simulink library "sm_car_lib"  (R2024a)
settings: Solver=VariableStepAuto  StartTime=0.0  StopTime=10.0  RelTol=1e-3
undefined symbols (not defined in the file or in its folder): acc_theta, accel_ramp_rate, circ_out, clr_upr, Control, hp1, hp2, hp3, hp_in_f_ua, hp_in_r_ua, hp_la_out, hp_ua_out, Init, Newton, opc_upr, radius_upr, Raphson, RDF_Rough_Road, rhs_hp, Scene, ShaftF, ShaftR, Vehicle, Visual, X, Y, Z
libraries: sm_lib x117, $bdroot x97, nesl_utility x36, simulink x17, fl_lib x6, sharedtransformsys x3, Brakes_Elements x2, Driver_Gamepad_Xbox x2, Multibody_Parts_Lib x2, sm_car_scene_track_mallory_park_obstacle x2, Testrig_4Post_Inputs x2, Aero_Coefficients x1
(part 4 of 7)

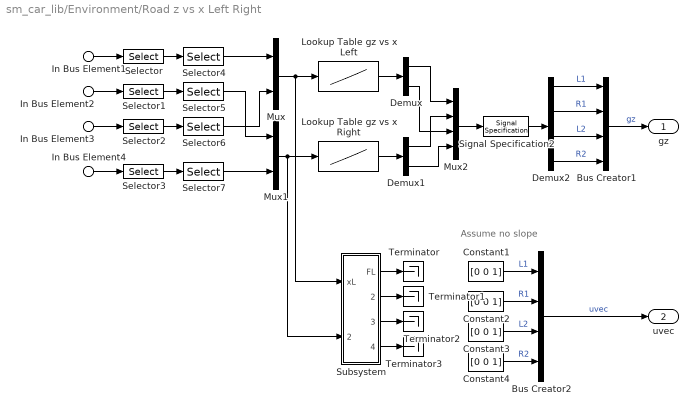
== system sm_car_lib/Environment/Road z vs x Left Right ==
  note: Assume no slope
  In Bus Element1 : Inport  PortName=Chassis  Element=WhlL1.xyz
  In Bus Element2 : Inport  PortName=Chassis  Element=WhlR1.xyz
  In Bus Element3 : Inport  PortName=Chassis  Element=WhlL2.xyz
  In Bus Element4 : Inport  PortName=Chassis  Element=WhlR2.xyz
  Bus Creator1 : BusCreator  Inputs=4
  Bus Creator2 : BusCreator  Inputs=4
  Constant{1..4} (4 alike) : Constant  Value=[0 0 1]
  Demux : Demux  Outputs=2
  Demux1 : Demux  Outputs=2
  Demux2 : Demux
  Lookup Table gz vs x Left : Lookup_n-D  NumberOfTableDimensions=1  BreakpointsForDimension1=dist_x_l  Table=height_z_l  InternalRulePriority=Speed  RndMeth=Simplest
  Lookup Table gz vs x Right : Lookup_n-D  NumberOfTableDimensions=1  BreakpointsForDimension1=dist_x_r  Table=height_z_r  InternalRulePriority=Speed  RndMeth=Simplest
  Mux : Mux  Inputs=2
  Mux1 : Mux  Inputs=2
  Mux2 : Mux
  Selector{,1..3} (4 alike) : Selector  InputPortWidth=3  IndexOptions=Index vector (dialog)  Indices=[1 2]  OutputSizes=1
  Selector{4..7} (4 alike) : Selector  InputPortWidth=2  IndexOptions=Index vector (dialog)  Indices=1  OutputSizes=1
  Signal Specification2 : SignalSpecification  Unit=m
  Subsystem : Subsystem
  Terminator{,1..3} (4 alike) : Terminator
  gz : Outport  VectorParamsAs1DForOutWhenUnconnected=off
  uvec : Outport  Port=2  VectorParamsAs1DForOutWhenUnconnected=off
  wires:
  Signal Specification2/1 -> Demux2/1
  In Bus Element3/1 -> Selector2/1
  In Bus Element1/1 -> Selector/1
  In Bus Element2/1 -> Selector1/1
  In Bus Element4/1 -> Selector3/1
  Selector/1 -> Selector4/1
  Selector1/1 -> Selector5/1
  Selector2/1 -> Selector6/1
  Selector3/1 -> Selector7/1
  Selector7/1 -> Mux1/2
  Selector6/1 -> Mux/2
  Selector5/1 -> Mux1/1
  Selector4/1 -> Mux/1
  Lookup Table gz vs x Right/1 -> Demux1/1
  Lookup Table gz vs x Left/1 -> Demux/1
  Demux/1 -> Mux2/1
  Demux1/1 -> Mux2/2
  Demux/2 -> Mux2/3
  Demux1/2 -> Mux2/4
  Mux2/1 -> Signal Specification2/1
  Mux1/1 -> Subsystem/2(xR), Lookup Table gz vs x Right/1
  Mux/1 -> Subsystem/1(xL), Lookup Table gz vs x Left/1
  Demux2/1 -> Bus Creator1/1  "L1"
  Demux2/2 -> Bus Creator1/2  "R1"
  Demux2/3 -> Bus Creator1/3  "L2"
  Demux2/4 -> Bus Creator1/4  "R2"
  Bus Creator1/1 -> gz/1  "gz"
  Constant1/1 -> Bus Creator2/1  "L1"
  Constant3/1 -> Bus Creator2/3  "L2"
  Constant2/1 -> Bus Creator2/2  "R1"
  Bus Creator2/1 -> uvec/1  "uvec"
  Constant4/1 -> Bus Creator2/4  "R2"
  Subsystem/1(FL) -> Terminator/1
  Subsystem/4(RR) -> Terminator3/1
  Subsystem/2(FR) -> Terminator1/1
  Subsystem/3(RL) -> Terminator2/1

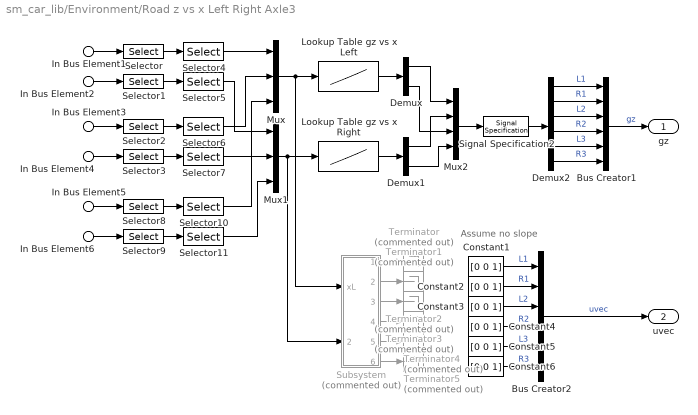
== system sm_car_lib/Environment/Road z vs x Left Right Axle3 ==
  note: Assume no slope
  In Bus Element1 : Inport  PortName=Chassis  Element=WhlL1.xyz
  In Bus Element2 : Inport  PortName=Chassis  Element=WhlR1.xyz
  In Bus Element3 : Inport  PortName=Chassis  Element=WhlL2.xyz
  In Bus Element4 : Inport  PortName=Chassis  Element=WhlR2.xyz
  In Bus Element5 : Inport  PortName=Chassis  Element=WhlL3.xyz
  In Bus Element6 : Inport  PortName=Chassis  Element=WhlR3.xyz
  Bus Creator1 : BusCreator  Inputs=6
  Bus Creator2 : BusCreator  Inputs=6
  Constant{1..6} (6 alike) : Constant  Value=[0 0 1]
  Demux : Demux  Outputs=2
  Demux1 : Demux  Outputs=2
  Demux2 : Demux  Outputs=6
  Lookup Table gz vs x Left : Lookup_n-D  NumberOfTableDimensions=1  BreakpointsForDimension1=dist_x_l  Table=height_z_l  InternalRulePriority=Speed  RndMeth=Simplest
  Lookup Table gz vs x Right : Lookup_n-D  NumberOfTableDimensions=1  BreakpointsForDimension1=dist_x_r  Table=height_z_r  InternalRulePriority=Speed  RndMeth=Simplest
  Mux : Mux  Inputs=3
  Mux1 : Mux  Inputs=3
  Mux2 : Mux
  Selector{,1..3,8..9} (6 alike) : Selector  InputPortWidth=3  IndexOptions=Index vector (dialog)  Indices=[1 2]  OutputSizes=1
  Selector{4..7,10..11} (6 alike) : Selector  InputPortWidth=2  IndexOptions=Index vector (dialog)  Indices=1  OutputSizes=1
  Signal Specification2 : SignalSpecification  Unit=m
  Subsystem : Subsystem  Commented=on
  Terminator{,1..5} (6 alike) : Terminator  Commented=on
  gz : Outport  VectorParamsAs1DForOutWhenUnconnected=off
  uvec : Outport  Port=2  VectorParamsAs1DForOutWhenUnconnected=off
  wires:
  Subsystem/3(L2) -> Terminator2/1
  Subsystem/2(R1) -> Terminator1/1
  Subsystem/4(R2) -> Terminator3/1
  Subsystem/1(L1) -> Terminator/1
  Constant4/1 -> Bus Creator2/4  "R2"
  Bus Creator2/1 -> uvec/1  "uvec"
  Constant2/1 -> Bus Creator2/2  "R1"
  Constant3/1 -> Bus Creator2/3  "L2"
  Constant1/1 -> Bus Creator2/1  "L1"
  Bus Creator1/1 -> gz/1  "gz"
  Demux2/4 -> Bus Creator1/4  "R2"
  Demux2/3 -> Bus Creator1/3  "L2"
  Demux2/2 -> Bus Creator1/2  "R1"
  Demux2/1 -> Bus Creator1/1  "L1"
  Mux/1 -> Lookup Table gz vs x Left/1, Subsystem/1(xL)
  Mux1/1 -> Lookup Table gz vs x Right/1, Subsystem/2(xR)
  Mux2/1 -> Signal Specification2/1
  Demux1/2 -> Mux2/4
  Demux/2 -> Mux2/3
  Demux1/1 -> Mux2/2
  Demux/1 -> Mux2/1
  Lookup Table gz vs x Left/1 -> Demux/1
  Lookup Table gz vs x Right/1 -> Demux1/1
  Selector4/1 -> Mux/1
  Selector5/1 -> Mux1/1
  Selector6/1 -> Mux/2
  Selector7/1 -> Mux1/2
  Selector3/1 -> Selector7/1
  Selector2/1 -> Selector6/1
  Selector1/1 -> Selector5/1
  Selector/1 -> Selector4/1
  In Bus Element4/1 -> Selector3/1
  In Bus Element2/1 -> Selector1/1
  In Bus Element1/1 -> Selector/1
  In Bus Element3/1 -> Selector2/1
  Signal Specification2/1 -> Demux2/1
  In Bus Element5/1 -> Selector8/1
  In Bus Element6/1 -> Selector9/1
  Selector8/1 -> Selector10/1
  Selector9/1 -> Selector11/1
  Selector10/1 -> Mux/3
  Selector11/1 -> Mux1/3
  Demux2/5 -> Bus Creator1/5  "L3"
  Demux2/6 -> Bus Creator1/6  "R3"
  Constant5/1 -> Bus Creator2/5  "L3"
  Constant6/1 -> Bus Creator2/6  "R3"
  Subsystem/5(L3) -> Terminator4/1
  Subsystem/6(R3) -> Terminator5/1

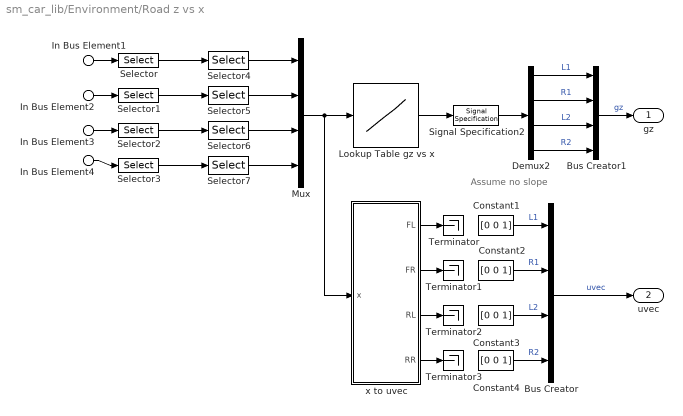
== system sm_car_lib/Environment/Road z vs x  ==
  note: Assume no slope
  In Bus Element1 : Inport  PortName=Chassis  Element=WhlL1.xyz
  In Bus Element2 : Inport  PortName=Chassis  Element=WhlR1.xyz
  In Bus Element3 : Inport  PortName=Chassis  Element=WhlL2.xyz
  In Bus Element4 : Inport  PortName=Chassis  Element=WhlR2.xyz
  Bus Creator : BusCreator  Inputs=4
  Bus Creator1 : BusCreator  Inputs=4
  Constant{1..4} (4 alike) : Constant  Value=[0 0 1]
  Demux2 : Demux
  Lookup Table gz vs x : Lookup_n-D  NumberOfTableDimensions=1  BreakpointsForDimension1=dist_x  Table=height_z  InternalRulePriority=Speed  RndMeth=Simplest
  Mux : Mux
  Selector{,1..3} (4 alike) : Selector  InputPortWidth=3  IndexOptions=Index vector (dialog)  Indices=[1 2]  OutputSizes=1
  Selector{4..7} (4 alike) : Selector  InputPortWidth=2  IndexOptions=Index vector (dialog)  Indices=1  OutputSizes=1
  Signal Specification2 : SignalSpecification  Unit=m
  Terminator{,1..3} (4 alike) : Terminator
  x to uvec : Subsystem
  gz : Outport  VectorParamsAs1DForOutWhenUnconnected=off
  uvec : Outport  Port=2  VectorParamsAs1DForOutWhenUnconnected=off
  wires:
  Lookup Table gz vs x/1 -> Signal Specification2/1
  Mux/1 -> x to uvec/1(x), Lookup Table gz vs x/1
  Selector4/1 -> Mux/1
  Selector5/1 -> Mux/2
  Selector6/1 -> Mux/3
  Selector7/1 -> Mux/4
  Selector3/1 -> Selector7/1
  Selector2/1 -> Selector6/1
  Selector1/1 -> Selector5/1
  Selector/1 -> Selector4/1
  In Bus Element4/1 -> Selector3/1
  In Bus Element2/1 -> Selector1/1
  In Bus Element1/1 -> Selector/1
  In Bus Element3/1 -> Selector2/1
  Demux2/3 -> Bus Creator1/3  "L2"
  Signal Specification2/1 -> Demux2/1
  Demux2/2 -> Bus Creator1/2  "R1"
  Demux2/1 -> Bus Creator1/1  "L1"
  Demux2/4 -> Bus Creator1/4  "R2"
  Bus Creator1/1 -> gz/1  "gz"
  Bus Creator/1 -> uvec/1  "uvec"
  Constant1/1 -> Bus Creator/1  "L1"
  x to uvec/1(FL) -> Terminator/1
  x to uvec/2(FR) -> Terminator1/1
  x to uvec/3(RL) -> Terminator2/1
  x to uvec/4(RR) -> Terminator3/1
  Constant2/1 -> Bus Creator/2  "R1"
  Constant3/1 -> Bus Creator/3  "L2"
  Constant4/1 -> Bus Creator/4  "R2"

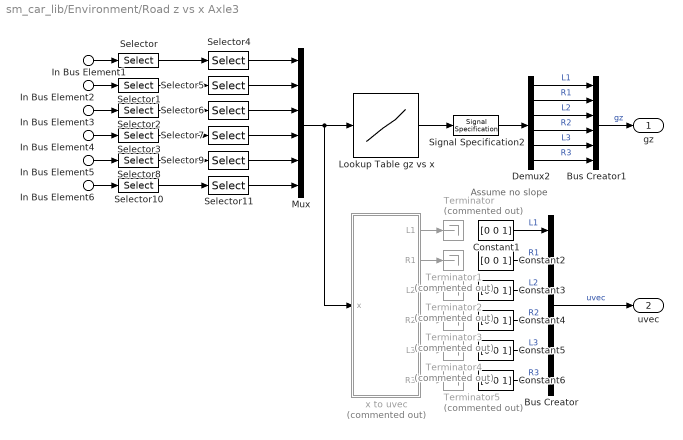
== system sm_car_lib/Environment/Road z vs x Axle3 ==
  note: Assume no slope
  In Bus Element1 : Inport  PortName=Chassis  Element=WhlL1.xyz
  In Bus Element2 : Inport  PortName=Chassis  Element=WhlR1.xyz
  In Bus Element3 : Inport  PortName=Chassis  Element=WhlL2.xyz
  In Bus Element4 : Inport  PortName=Chassis  Element=WhlR2.xyz
  In Bus Element5 : Inport  PortName=Chassis  Element=WhlL3.xyz
  In Bus Element6 : Inport  PortName=Chassis  Element=WhlR3.xyz
  Bus Creator : BusCreator  Inputs=6
  Bus Creator1 : BusCreator  Inputs=6
  Constant{1..6} (6 alike) : Constant  Value=[0 0 1]
  Demux2 : Demux  Outputs=6
  Lookup Table gz vs x : Lookup_n-D  NumberOfTableDimensions=1  BreakpointsForDimension1=dist_x  Table=height_z  InternalRulePriority=Speed  RndMeth=Simplest
  Mux : Mux  Inputs=6
  Selector{,1..3,8,10} (6 alike) : Selector  InputPortWidth=3  IndexOptions=Index vector (dialog)  Indices=[1 2]  OutputSizes=1
  Selector{4..7,9,11} (6 alike) : Selector  InputPortWidth=2  IndexOptions=Index vector (dialog)  Indices=1  OutputSizes=1
  Signal Specification2 : SignalSpecification  Unit=m
  Terminator{,1..5} (6 alike) : Terminator  Commented=on
  x to uvec : Subsystem  Commented=on
  gz : Outport  VectorParamsAs1DForOutWhenUnconnected=off
  uvec : Outport  Port=2  VectorParamsAs1DForOutWhenUnconnected=off
  wires:
  Constant4/1 -> Bus Creator/4  "R2"
  Constant3/1 -> Bus Creator/3  "L2"
  Constant2/1 -> Bus Creator/2  "R1"
  x to uvec/4(R2) -> Terminator3/1
  x to uvec/3(L2) -> Terminator2/1
  x to uvec/2(R1) -> Terminator1/1
  x to uvec/1(L1) -> Terminator/1
  Constant1/1 -> Bus Creator/1  "L1"
  Bus Creator/1 -> uvec/1  "uvec"
  Bus Creator1/1 -> gz/1  "gz"
  Demux2/4 -> Bus Creator1/4  "R2"
  Demux2/1 -> Bus Creator1/1  "L1"
  Demux2/2 -> Bus Creator1/2  "R1"
  Signal Specification2/1 -> Demux2/1
  Demux2/3 -> Bus Creator1/3  "L2"
  In Bus Element3/1 -> Selector2/1
  In Bus Element1/1 -> Selector/1
  In Bus Element2/1 -> Selector1/1
  In Bus Element4/1 -> Selector3/1
  Selector/1 -> Selector4/1
  Selector1/1 -> Selector5/1
  Selector2/1 -> Selector6/1
  Selector3/1 -> Selector7/1
  Selector7/1 -> Mux/4
  Selector6/1 -> Mux/3
  Selector5/1 -> Mux/2
  Selector4/1 -> Mux/1
  Mux/1 -> Lookup Table gz vs x/1, x to uvec/1(x)
  Lookup Table gz vs x/1 -> Signal Specification2/1
  Selector8/1 -> Selector9/1
  In Bus Element5/1 -> Selector8/1
  Selector9/1 -> Mux/5
  Selector11/1 -> Mux/6
  In Bus Element6/1 -> Selector10/1
  Selector10/1 -> Selector11/1
  Constant5/1 -> Bus Creator/5  "L3"
  Constant6/1 -> Bus Creator/6  "R3"
  Demux2/5 -> Bus Creator1/5  "L3"
  Demux2/6 -> Bus Creator1/6  "R3"
  x to uvec/5(L3) -> Terminator4/1
  x to uvec/6(R3) -> Terminator5/1

== system sm_car_lib/Environment/STL Geometry ==
  Geometry : sm_lib/Body Elements/File Solid  ExtGeomFileName=Bar1_Default_sldprt.STL  UnitType=Custom  ExtGeomFileUnits=m  StepReaderType=HEX  ExportConvexHullGeometry=off  InertiaType=Custom  BasedOnType=DensityFromFile  Density=1000  DensityUnits=kg/m^3  Mass=1  MassUnits=kg  CenterOfMass=[0 0 0]  CenterOfMassUnits=m  MomentsOfInertia=[1 1 1]  MomentsOfInertiaUnits=kg*m^2  ProductsOfInertia=[0 0 0]  ProductsOfInertiaUnits=kg*m^2  GraphicType=FromGeometry  MarkerShape=Sphere  MarkerSize=10  GraphicVisPropType=SimpleVisualProperties  GraphicDiffuseColor=stl_clr  GraphicOpacity=stl_opc  GraphicSpecularColor=[0.5 0.5 0.5 1.0]  GraphicAmbientColor=[0.15 0.15 0.15 1.0]  GraphicEmissiveColor=[0.0 0.0 0.0 1.0]  GraphicShininess=75  DoExposeReferenceFrame=on  SerializedFrames=<Frames/>
  Transform Geometry : sm_lib/Frames and Transforms/Rigid Transform  RotationMethod=RotationSequence  FollAlignAxisA=+X  BaseAlignAxisA=+Y  FollAlignAxisB=+Y  BaseAlignAxisB=+Z  RotationStandardAxis=+Z  RotationAngle=0  RotationAngleUnits=rad  RotationArbitraryAxis=[0 0 1]  RotationSequenceAxes=FollowerAxes  RotationSequence=ZYX  RotationSequenceAngles=[stl_yaw stl_pitch stl_roll]  RotationSequenceAnglesUnits=rad  RotationMatrix=[1 0 0; 0 1 0; 0 0 1]  Quaternion=[1 0 0 0]  TranslationMethod=Cartesian  TranslationCartesianOffset=[stl_x stl_y stl_z]  TranslationCartesianOffsetUnits=m  TranslationStandardAxis=+Z  TranslationStandardOffset=0  TranslationStandardOffsetUnits=m  TranslationROffset=0  TranslationROffsetUnits=m  TranslationThetaOffset=0  TranslationThetaOffsetUnits=deg  TranslationZOffset=0  TranslationZOffsetUnits=m
  W : PMIOPort  Side=Right
  connections:
  Geometry/RConn1 -- Transform Geometry/RConn1
  Transform Geometry/LConn1 -- W/RConn1

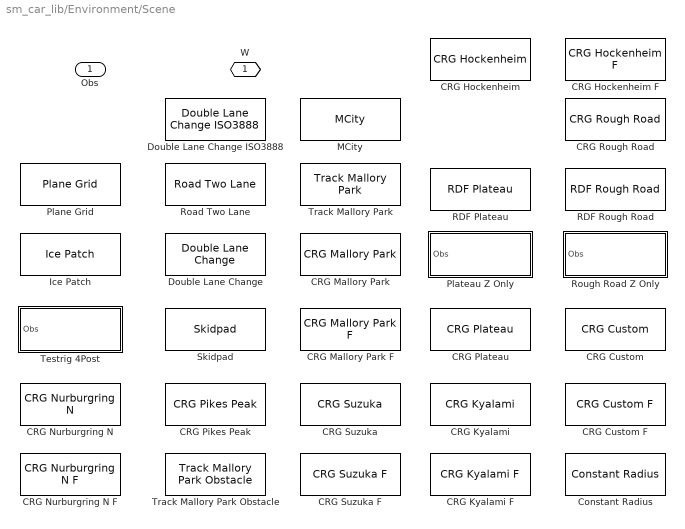
== system sm_car_lib/Environment/Scene ==
  CRG Custom : sm_car_scene_crg_custom/CRG Custom  VariantControl=CRG_Custom  geometry=Scene.CRG_Custom.Geometry
  CRG Custom F : sm_car_scene_crg_custom_f/CRG Custom F  VariantControl=CRG_Custom_F  geometry=Scene.CRG_Custom_F.Geometry
  CRG Hockenheim : sm_car_scene_crg_hockenheim/CRG Hockenheim  VariantControl=CRG_Hockenheim  geometry=Scene.CRG_Hockenheim.Geometry
  CRG Hockenheim F : sm_car_scene_crg_hockenheim_f/CRG Hockenheim F  VariantControl=CRG_Hockenheim_F  geometry=Scene.CRG_Hockenheim_F.Geometry
  CRG Kyalami : sm_car_scene_crg_kyalami/CRG Kyalami  VariantControl=CRG_Kyalami  geometry=Scene.CRG_Kyalami.Geometry
  CRG Kyalami F : sm_car_scene_crg_kyalami_f/CRG Kyalami F  VariantControl=CRG_Kyalami_F  geometry=Scene.CRG_Kyalami_F.Geometry
  CRG Mallory Park : sm_car_scene_crg_mallory_park/CRG Mallory Park  VariantControl=CRG_Mallory_Park  geometry=Scene.CRG_Mallory_Park.Geometry
  CRG Mallory Park F : sm_car_scene_crg_mallory_park_f/CRG Mallory Park F  VariantControl=CRG_Mallory_Park_F  geometry=Scene.CRG_Mallory_Park_F.Geometry
  CRG Nurburgring N : sm_car_scene_crg_nurburgring_n/CRG Nurburgring N  VariantControl=CRG_Nurburgring_N  geometry=Scene.CRG_Nurburgring_N.Geometry
  CRG Nurburgring N F : sm_car_scene_crg_nurburgring_n_f/CRG Nurburgring N F  VariantControl=CRG_Nurburgring_N_F  geometry=Scene.CRG_Nurburgring_N_F.Geometry
  CRG Pikes Peak : sm_car_scene_crg_pikes_peak/CRG Pikes Peak  VariantControl=CRG_Pikes_Peak  geometry=Scene.CRG_Pikes_Peak.Geometry
  CRG Plateau : sm_car_scene_crg_plateau/CRG Plateau  VariantControl=CRG_Plateau  geometry=Scene.CRG_Plateau.Geometry
  CRG Rough Road : sm_car_scene_crg_rough_road/CRG Rough Road  VariantControl=CRG_Rough_Road  geometry=Scene.CRG_Rough_Road.Geometry
  CRG Suzuka : sm_car_scene_crg_suzuka/CRG Suzuka  VariantControl=CRG_Suzuka  geometry=Scene.CRG_Suzuka.Geometry
  CRG Suzuka F : sm_car_scene_crg_suzuka_f/CRG Suzuka F  VariantControl=CRG_Suzuka_F  geometry=Scene.CRG_Suzuka_F.Geometry
  Constant Radius : sm_car_scene_constant_radius_cl/Constant Radius  VariantControl=Constant_Radius  circ_in=Scene.Constant_Radius_CL.Circle_Inner  circ_out=Scene.Constant_Radius_CL.Circle_Outer  plane=Scene.Constant_Radius_CL.Plane
  Double Lane Change : sm_car_scene_double_lane_change/Double Lane Change  VariantControl=Double_Lane_Change  road=Scene.Double_Lane_Change.Road  dashes=Scene.Double_Lane_Change.Dashes  cones=Scene.Double_Lane_Change.Cones
  Double Lane Change ISO3888 : sm_car_scene_double_lane_change_iso3888/Double Lane Change ISO3888  VariantControl=Double_Lane_Change_ISO3888  road=Scene.Double_Lane_Change_ISO3888.Road  dashes=Scene.Double_Lane_Change_ISO3888.Dashes  cones=Scene.Double_Lane_Change_ISO3888.Cones
  Ice Patch : sm_car_scene_ice_patch/Ice Patch  VariantControl=Ice_Patch  plane=Scene.Ice_Patch.Plane  grid=Scene.Ice_Patch.Grid  ice=Scene.Ice_Patch.Ice
  MCity : sm_car_scene_mcity/MCity  VariantControl=MCity  geometry=Scene.MCity.Geometry
  Plane Grid : sm_car_scene_plane_grid/Plane Grid  VariantControl=Plane_Grid  plane=Scene.Plane_Grid.Plane  grid=Scene.Plane_Grid.Grid
  Plateau Z Only : Subsystem  VariantControl=Plateau_Z_Only  mask{RDF_Polyline=Scene.RDF_Plateau}
      mask prompts: RDF_Polyline "RDF Polyline (structure)"
  RDF Plateau : sm_car_scene_rdf_plateau/RDF Plateau  VariantControl=RDF_Plateau  RDF_Polyline=Scene.RDF_Plateau
  RDF Rough Road : sm_car_scene_rdf_rough_road/RDF Rough Road  VariantControl=RDF_Rough_Road  RDF_Polyline=Scene.RDF_Rough_Road
  Road Two Lane : sm_car_scene_road_two_lane/Road Two Lane  VariantControl=Road_Two_Lane  road=Scene.Road_Two_Lane.Road  dashes=Scene.Road_Two_Lane.Dashes
  Rough Road Z Only : Subsystem  VariantControl=Rough_Road_Z_Only  mask{RDF_Polyline=Scene.RDF_Rough_Road}
      mask prompts: RDF_Polyline "RDF Polyline (structure)"
  Skidpad : sm_car_scene_skidpad/Skidpad  VariantControl=Skidpad  circ_in=Scene.Skidpad.Circle_Inner  circ_out=Scene.Skidpad.Circle_Outer  plane=Scene.Skidpad.Plane
  Testrig 4Post : Subsystem  VariantControl=Testrig_4_Post
  Track Mallory Park : sm_car_scene_track_mallory_park/Track Mallory Park  VariantControl=Track_Mallory_Park  track=Scene.Mallory_Park.Track
  Track Mallory Park Obstacle : sm_car_scene_track_mallory_park_obstacle/Track Mallory Park Obstacle  VariantControl=Track_Mallory_Park_Obstacle  scene_data=Scene.Mallory_Park_Obstacle
  W : PMIOPort  Side=Left
  Obs : Outport  VectorParamsAs1DForOutWhenUnconnected=off

== system sm_car_lib/Environment/Stripe Ring ==
  Solid : sm_lib/Body Elements/Extruded Solid  ExtrusionType=General  PolygonNumSides=3  PolygonOuterRadius=1  PolygonOuterRadiusUnits=m  ExportEntireGeometry=off  ExtrusionCrossSection=xy_data_circ  ExtrusionCrossSectionUnits=m  ExportConvexHullGeometry=off  ExtrusionLength=circ_h  ExtrusionLengthUnits=m  InertiaType=CalculateFromGeometry  BasedOnType=Density  Density=1000  DensityUnits=kg/m^3  Mass=1  MassUnits=kg  CenterOfMass=[0 0 0]  CenterOfMassUnits=m  MomentsOfInertia=[1 1 1]  MomentsOfInertiaUnits=kg*m^2  ProductsOfInertia=[1 1 1]  ProductsOfInertiaUnits=kg*m^2  GraphicType=FromGeometry  MarkerShape=Sphere  MarkerSize=10  GraphicVisPropType=SimpleVisualProperties  GraphicDiffuseColor=[1.0 1.0 0.8]  GraphicOpacity=1.0  GraphicSpecularColor=[0.5 0.5 0.5 1.0]  GraphicAmbientColor=[0.15 0.15 0.15 1.0]  GraphicEmissiveColor=[0.0 0.0 0.0 1.0]  GraphicShininess=75  DoExposeReferenceFrame=on  SerializedFrames=<Frames/>
  W : PMIOPort  Side=Right
  connections:
  Solid/RConn1 -- W/RConn1

== system sm_car_lib/Environment/Track Extrusion ==
  Track : sm_lib/Body Elements/Extruded Solid  ExtrusionType=General  PolygonNumSides=3  PolygonOuterRadius=1  PolygonOuterRadiusUnits=m  ExportEntireGeometry=off  ExtrusionCrossSection=track_extr_data  ExtrusionCrossSectionUnits=m  ExportConvexHullGeometry=off  ExtrusionLength=track_h  ExtrusionLengthUnits=m  InertiaType=CalculateFromGeometry  BasedOnType=Density  Density=1000  DensityUnits=kg/m^3  Mass=1  MassUnits=kg  CenterOfMass=[0 0 0]  CenterOfMassUnits=m  MomentsOfInertia=[1 1 1]  MomentsOfInertiaUnits=kg*m^2  ProductsOfInertia=[0 0 0]  ProductsOfInertiaUnits=kg*m^2  GraphicType=FromGeometry  MarkerShape=Sphere  MarkerSize=10  GraphicVisPropType=SimpleVisualProperties  GraphicDiffuseColor=track_clr  GraphicOpacity=track_opc  GraphicSpecularColor=[0.5 0.5 0.5 1.0]  GraphicAmbientColor=[0.15 0.15 0.15 1.0]  GraphicEmissiveColor=[0.0 0.0 0.0 1.0]  GraphicShininess=75  DoExposeReferenceFrame=on  SerializedFrames=<Frames/>
  Transform Track : sm_lib/Frames and Transforms/Rigid Transform  RotationMethod=StandardAxis  FollAlignAxisA=+X  BaseAlignAxisA=+Y  FollAlignAxisB=+Y  BaseAlignAxisB=+Z  RotationStandardAxis=+Z  RotationAngle=track_yaw  RotationAngleUnits=rad  RotationArbitraryAxis=[0 0 1]  RotationSequenceAxes=FollowerAxes  RotationSequence=XYX  RotationSequenceAngles=[0 0 0]  RotationSequenceAnglesUnits=deg  RotationMatrix=[1 0 0; 0 1 0; 0 0 1]  Quaternion=[1 0 0 0]  TranslationMethod=Cartesian  TranslationCartesianOffset=[track_x track_y track_z-track_h/2]  TranslationCartesianOffsetUnits=m  TranslationStandardAxis=+Z  TranslationStandardOffset=0  TranslationStandardOffsetUnits=m  TranslationROffset=0  TranslationROffsetUnits=m  TranslationThetaOffset=0  TranslationThetaOffsetUnits=deg  TranslationZOffset=0  TranslationZOffsetUnits=m
  W : PMIOPort  Side=Right
  connections:
  Transform Track/LConn1 -- W/RConn1
  Track/RConn1 -- Transform Track/RConn1

== system sm_car_lib/Inputs/Control Bus ==
  Brake : Subsystem  mask{brake_on_time=10}
      mask prompts: brake_on_time "Brake On Time (sec)"
      mask TypeOptions brake_on_time: Step/Time
  Bus Creator : BusCreator  Inputs=4
  Bus Creator1 : BusCreator  Inputs=4
  Power Control : Subsystem
  Spring Damper : Subsystem
  Susp : Subsystem
  Torque Input : Subsystem  mask{popup_torque_input=Low Torque, Rear}
      mask prompts: popup_torque_input "Maneuver Torque"
      mask init:
      | if (popup_torque_input == 1)
      |     torque_ra = 200*2*2*2;
      |     torque_fa = 0;
      | elseif (popup_torque_input == 2)
      |     torque_ra = 0;
      |     torque_fa = 200*2*2*2;
      | elseif (popup_torque_input == 3)
      |     torque_ra = 200*2;
      |     torque_fa = 0;
      | elseif (popup_torque_input == 4)
      |     torque_ra = 0;
      |     torque_fa = 200*2;
      | elseif (popup_torque_input == 5)
      |     torque_ra = 0;
      |     torque_fa = 0;
      | end
      mask TypeOptions popup_torque_input: Full Torque, Rear | Full Torque, Front | Low Torque, Rear | Low Torque, Front | None
  CtrlBus : Outport  VectorParamsAs1DForOutWhenUnconnected=off
  wires:
  Susp/1(SuspA1) -> Bus Creator/3
  Susp/2(SuspA2) -> Bus Creator/4
  Bus Creator1/1 -> CtrlBus/1  "CtrlBus"
  Spring Damper/1(Damper) -> Bus Creator/2
  Spring Damper/2(Spring) -> Bus Creator/1
  Brake/1(Brk) -> Bus Creator1/1
  Torque Input/1(Driveline) -> Bus Creator1/4
  Bus Creator/1 -> Bus Creator1/2  "Chassis"
  Power Control/1(Power) -> Bus Creator1/3

== system sm_car_lib/Inputs/Control Bus Axle3 ==
  Brake : Subsystem  mask{brake_on_time=10}
      mask prompts: brake_on_time "Brake On Time (sec)"
      mask TypeOptions brake_on_time: Step/Time
  Bus Creator : BusCreator  Inputs=7
  Spring Damper : Subsystem
  SuspF : Subsystem
  Torque Input : Subsystem  mask{popup_torque_input=Low Torque, Rear}
      mask prompts: popup_torque_input "Maneuver Torque"
      mask init: same as sm_car_lib/Inputs/Control Bus/Torque Input
      mask TypeOptions popup_torque_input: Full Torque, Rear | Full Torque, Front | Low Torque, Rear | Low Torque, Front | None
  CtrlBus : Outport  VectorParamsAs1DForOutWhenUnconnected=off
  wires:
  Torque Input/1(Driveline) -> Bus Creator/7
  Brake/1(Brk) -> Bus Creator/1
  Spring Damper/1(Spring) -> Bus Creator/2
  Spring Damper/2(Damper) -> Bus Creator/3
  Bus Creator/1 -> CtrlBus/1  "CtrlBus"
  SuspF/2(SuspA2) -> Bus Creator/5
  SuspF/1(SuspA1) -> Bus Creator/4
  SuspF/3(SuspA3) -> Bus Creator/6

== system sm_car_lib/Inputs/DrvBus ==
  Accel : Subsystem  mask{brake_on_time=10}
      mask prompts: brake_on_time "Brake On Time (sec)"
      mask TypeOptions brake_on_time: Step/Time
  Brake : Subsystem  mask{brake_on_time=10}
      mask prompts: brake_on_time "Brake On Time (sec)"
      mask TypeOptions brake_on_time: Step/Time
  Bus Creator : BusCreator  Inputs=3
  Steer Input : Subsystem  mask{popup_steer_input=Sequence}
      mask prompts: popup_steer_input "Steer Input"
      mask TypeOptions popup_steer_input: Straight | Step | Sequence | Lane Change
  Terminator : Terminator
  Torque Input : Subsystem  mask{popup_torque_input=Full Torque}
      mask prompts: popup_torque_input "Maneuver Torque"
      mask init:
      | if (popup_torque_input == 1)
      |     rPedalValue = 1;
      | elseif (popup_torque_input == 2)
      |     rPedalValue = 0.25;
      | elseif (popup_torque_input == 3)
      |     rPedalValue = 0;
      | end
      mask TypeOptions popup_torque_input: Full Torque | Low Torque | None
  Out1 : Outport  VectorParamsAs1DForOutWhenUnconnected=off
  wires:
  Steer Input/1(DrvBus) -> Bus Creator/3
  Bus Creator/1 -> Out1/1
  Brake/1(Brk) -> Bus Creator/2
  Torque Input/1(rAccelPedal) -> Bus Creator/1
  Accel/1(Brk) -> Terminator/1

== system sm_car_lib/Inputs/Road Bus ==
  Bus Creator1 : BusCreator  Inputs=3
  Bus Creator2 : BusCreator  Inputs=3
  Bus Creator3 : BusCreator  Inputs=6
  Constant{1..3,5} (4 alike) : Constant  Value=[0 0 0 0 0 0 0 0]
  Constant{4,6..10} (6 alike) : Constant  Value=0
  Ground : Subsystem
  None : Subsystem  VariantControl=None
  Out1 : Outport  VectorParamsAs1DForOutWhenUnconnected=off
  wires:
  None/1(gz) -> Ground/1(gz)
  None/2(uvec) -> Ground/2(uvec)
  Constant5/1 -> Ground/3(TyreScaling FL)  "TyreScalingFL"
  Constant1/1 -> Ground/4(TyreScaling FR)  "TyreScalingFR"
  Constant2/1 -> Ground/5(TyreScaling RL)  "TyreScalingRL"
  Constant3/1 -> Ground/6(TyreScaling RR)  "TyreScalingRR"
  Constant6/1 -> Bus Creator1/2  "fy"
  Constant7/1 -> Bus Creator1/3  "fz"
  Constant4/1 -> Bus Creator1/1  "fx"
  Bus Creator1/1 -> Bus Creator3/5  "fWindCar"
  Constant8/1 -> Bus Creator2/1  "fx"
  Constant10/1 -> Bus Creator2/3  "fz"
  Constant9/1 -> Bus Creator2/2  "fy"
  Bus Creator2/1 -> Bus Creator3/6  "fWindTrailer"
  Ground/1(L1) -> Bus Creator3/1
  Ground/2(R1) -> Bus Creator3/2
  Ground/3(L2) -> Bus Creator3/3
  Ground/4(R2) -> Bus Creator3/4
  Bus Creator3/1 -> Out1/1

== system sm_car_lib/Maneuver/Check ==
  l : Inport
  v : Inport  Port=2
  Bus Selector : BusSelector  OutputSignals=World.vx,World.vy  OutputAsBus=on
  Bus Selector1 : BusSelector  OutputSignals=Reference.latdev,Reference.dist
  End Lap : Constant  Value=0.2
  Lateral Deviation Threshold : Constant  Value=lat_dev_threshold
  Less Than : RelationalOperator  Operator=<  OutDataTypeStr=boolean  RndMeth=Simplest  InputSameDT=off
  Less Than1 : RelationalOperator  Operator=>  OutDataTypeStr=boolean  ZeroCross=off  RndMeth=Simplest  InputSameDT=off
  Less Than2 : RelationalOperator  Operator=<  OutDataTypeStr=boolean  ZeroCross=off  RndMeth=Simplest  InputSameDT=off
  Less Than3 : RelationalOperator  Operator=>  OutDataTypeStr=boolean  RndMeth=Simplest  InputSameDT=off
  Max Speed Threshold : Constant  Value=max_speed
  Product{,1..3} (4 alike) : Product
  Start Checking : Step  Time=start_check_time  SampleTime=0  ZeroCross=off
  Start Checking End Lap : Step  Time=start_check_time_end_lap  SampleTime=0  ZeroCross=off
  Start Checking Lat Dev : Step  Time=start_check_time_ld  SampleTime=0  ZeroCross=off
  Start Checking Max Speed : Step  Time=start_check_time_max_speed  SampleTime=0  ZeroCross=off
  Stop Threshold : Constant  Value=stop_speed
  Sum : Sum  Inputs=++++
  Vel in xy plane : Fcn  Expr=sqrt(u(1)^2+u(2)^2)
  Stop : Outport  VectorParamsAs1DForOutWhenUnconnected=off
  wires:
  Less Than/1 -> Product/1
  Stop Threshold/1 -> Less Than/2
  v/1 -> Bus Selector/1
  Start Checking/1 -> Product/2
  Product/1 -> Sum/1
  Bus Selector/1 -> Vel in xy plane/1
  Vel in xy plane/1 -> Less Than/1, Less Than3/1  "speed"
  l/1 -> Bus Selector1/1
  Bus Selector1/1 -> Less Than1/1  "<latdev>"
  Lateral Deviation Threshold/1 -> Less Than1/2
  Less Than1/1 -> Product1/1
  Start Checking Lat Dev/1 -> Product1/2
  Sum/1 -> Stop/1
  Product1/1 -> Sum/3
  End Lap/1 -> Less Than2/2
  Bus Selector1/2 -> Less Than2/1  "<dist>"
  Less Than2/1 -> Product2/1
  Start Checking End Lap/1 -> Product2/2
  Product2/1 -> Sum/4
  Start Checking Max Speed/1 -> Product3/2
  Less Than3/1 -> Product3/1
  Max Speed Threshold/1 -> Less Than3/2
  Product3/1 -> Sum/2

== system sm_car_lib/Outputs/VehBus ==
  Brakes : Subsystem
  Bus Creator : BusCreator  Inputs=3
  DoF : $bdroot/Body/Body to World  Init=Init.Chassis  SpecifyPosTarget=on
  Reference Frame : sm_lib/Frames and Transforms/Reference Frame
  Solver Configuration : nesl_utility/Solver Configuration  PhysicalDomain=network_engine_domain  SubClassName=solver  LeftPortType=input  RightPortType=generic  Tones=[]  Harmonics=[]  SimulateNoise=off  Profile=off  UseLocalSampling=off  EnableSwitchedLinearOptims=on  FrequencyDomain=off  UseCCode=off  RelTol=0.001  AbsTol=1e-06  MinStep=1e-09  ToWorkspace=off  RevertToSquareIcSolve=off  NumHomotopyIterations=100  PhasorMode=off  PhasorModeNumHarmonics=1  ConsistencySolver=NEWTON_FTOL  IndexReductionMethod=DerivativeReplacement  DoDC=off  ResidualTolerance=1e-09  ConsistencyTolSource=GLOBAL  ConsistencyAbsTol=0.001  ConsistencyRelTol=0.001  ConsistencyTolFactor=0.001  UseLocalSolver=off  LocalSolverChoice=NE_BACKWARD_EULER_ADVANCER  ResolveIndetEquations=on  FunctionEvalNumThread=1  LocalSolverSampleTime=0.001  DoFixedCost=off  MaxNonlinIter=3  MaxModeIter=2  ComputeImpulses=off  ImpulseIterations=2  LinearAlgebra=auto  LinearAlgebraNumThread=0  EquationFormulation=NE_TIME_EF  DelaysMemoryBudget=1024  AutomaticFiltering=on  FilteringTimeConstant=0.001  PartitionStorageMethod=AS_NEEDED  PartitionMemoryBudget=1024  PartitionMethod=FAST  MultibodyUseLocalSolver=off  MultibodyLocalSolverChoice=ODE1  MultibodyLocalSolverSampleTime=0.001
  Subsystem : Subsystem
  World Frame : sm_lib/Frames and Transforms/World Frame
  VehBus : Outport  VectorParamsAs1DForOutWhenUnconnected=off
  wires:
  Brakes/1(Brakes) -> Bus Creator/3  "Brakes"
  DoF/1 -> Bus Creator/2  "World"
  Subsystem/1(Chassis) -> Bus Creator/1  "Chassis"
  Bus Creator/1 -> VehBus/1  "VehBus"
  connections:
  World Frame/RConn1 -- DoF/LConn1 -- Solver Configuration/RConn1 -- Subsystem/LConn1
  DoF/RConn1 -- Reference Frame/RConn1

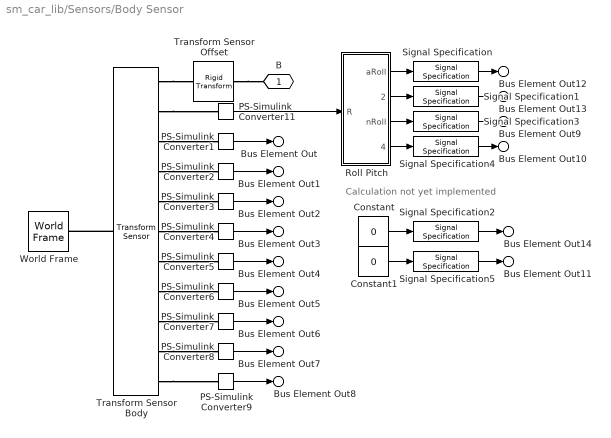
== system sm_car_lib/Sensors/Body Sensor ==
  note: Calculation not yet implemented
  Constant : Constant  Value=0
  Constant1 : Constant  Value=0
  PS-Simulink Converter1 : nesl_utility/PS-Simulink Converter  PhysicalDomain=network_engine_domain  SubClassName=ps_output  LeftPortType=input  RightPortType=output  PseudoPeriodic=off  Frequencies=[]  VectorFormat=1-D array  Unit=m  AffineConversion=off
  PS-Simulink Converter11 : nesl_utility/PS-Simulink Converter  PhysicalDomain=network_engine_domain  SubClassName=ps_output  LeftPortType=input  RightPortType=output  PseudoPeriodic=off  Frequencies=[]  VectorFormat=1-D array  Unit=1  AffineConversion=off
  PS-Simulink Converter2 : nesl_utility/PS-Simulink Converter  PhysicalDomain=network_engine_domain  SubClassName=ps_output  LeftPortType=input  RightPortType=output  PseudoPeriodic=off  Frequencies=[]  VectorFormat=1-D array  Unit=m  AffineConversion=off
  PS-Simulink Converter3 : nesl_utility/PS-Simulink Converter  PhysicalDomain=network_engine_domain  SubClassName=ps_output  LeftPortType=input  RightPortType=output  PseudoPeriodic=off  Frequencies=[]  VectorFormat=1-D array  Unit=m  AffineConversion=off
  PS-Simulink Converter4 : nesl_utility/PS-Simulink Converter  PhysicalDomain=network_engine_domain  SubClassName=ps_output  LeftPortType=input  RightPortType=output  PseudoPeriodic=off  Frequencies=[]  VectorFormat=1-D array  Unit=m/s  AffineConversion=off
  PS-Simulink Converter5 : nesl_utility/PS-Simulink Converter  PhysicalDomain=network_engine_domain  SubClassName=ps_output  LeftPortType=input  RightPortType=output  PseudoPeriodic=off  Frequencies=[]  VectorFormat=1-D array  Unit=m/s  AffineConversion=off
  PS-Simulink Converter6 : nesl_utility/PS-Simulink Converter  PhysicalDomain=network_engine_domain  SubClassName=ps_output  LeftPortType=input  RightPortType=output  PseudoPeriodic=off  Frequencies=[]  VectorFormat=1-D array  Unit=m/s  AffineConversion=off
  PS-Simulink Converter7 : nesl_utility/PS-Simulink Converter  PhysicalDomain=network_engine_domain  SubClassName=ps_output  LeftPortType=input  RightPortType=output  PseudoPeriodic=off  Frequencies=[]  VectorFormat=1-D array  Unit=m/s^2  AffineConversion=off
  PS-Simulink Converter8 : nesl_utility/PS-Simulink Converter  PhysicalDomain=network_engine_domain  SubClassName=ps_output  LeftPortType=input  RightPortType=output  PseudoPeriodic=off  Frequencies=[]  VectorFormat=1-D array  Unit=m/s^2  AffineConversion=off
  PS-Simulink Converter9 : nesl_utility/PS-Simulink Converter  PhysicalDomain=network_engine_domain  SubClassName=ps_output  LeftPortType=input  RightPortType=output  PseudoPeriodic=off  Frequencies=[]  VectorFormat=1-D array  Unit=m/s^2  AffineConversion=off
  Roll Pitch : Subsystem
  Signal Specification : SignalSpecification  Unit=rad
  Signal Specification1 : SignalSpecification  Unit=rad
  Signal Specification2 : SignalSpecification  Unit=rad
  Signal Specification3 : SignalSpecification  Unit=rad/s
  Signal Specification4 : SignalSpecification  Unit=rad/s
  Signal Specification5 : SignalSpecification  Unit=rad/s
  Transform Sensor Offset : sm_lib/Frames and Transforms/Rigid Transform  RotationMethod=None  FollAlignAxisA=+X  BaseAlignAxisA=+Y  FollAlignAxisB=+Y  BaseAlignAxisB=+Z  RotationStandardAxis=+Z  RotationAngle=0.0  RotationAngleUnits=deg  RotationArbitraryAxis=[0 0 1]  RotationSequenceAxes=FollowerAxes  RotationSequence=XYX  RotationSequenceAngles=[0 0 0]  RotationSequenceAnglesUnits=deg  RotationMatrix=[1 0 0; 0 1 0; 0 0 1]  Quaternion=[1 0 0 0]  TranslationMethod=Cartesian  TranslationCartesianOffset=offset_body_sensor  TranslationCartesianOffsetUnits=m  TranslationStandardAxis=+Z  TranslationStandardOffset=0  TranslationStandardOffsetUnits=m  TranslationROffset=0  TranslationROffsetUnits=m  TranslationThetaOffset=0  TranslationThetaOffsetUnits=deg  TranslationZOffset=0  TranslationZOffsetUnits=m
  Transform Sensor Body : sm_lib/Frames and Transforms/Transform Sensor  MeasurementFrame=NonRotatingFollower  RotationSequence=XYX  SenseAngle=off  SenseAxis=off  SenseQ=off  SenseR=on  SenseRotationSequence=off  SenseOmegaX=off  SenseOmegaY=off  SenseOmegaZ=off  SenseOmega=off  SenseQDot=off  SenseRDot=off  SenseRotationSequenceDot=off  SenseAlphaX=off  SenseAlphaY=off  SenseAlphaZ=off  SenseAlpha=off  SenseQDDot=off  SenseRDDot=off  SenseX=on  SenseY=on  SenseZ=on  SenseXYZ=off  SenseRad=off  SenseAzim=off  SenseDist=off  SenseInc=off  SenseXDot=on  SenseYDot=on  SenseZDot=on  SenseXYZDot=off  SenseRadDot=off  SenseAzimDot=off  SenseDistDot=off  SenseIncDot=off  SenseXDDot=on  SenseYDDot=on  SenseZDDot=on  SenseXYZDDot=off  SenseRadDDot=off  SenseAzimDDot=off  SenseDistDDot=off  SenseIncDDot=off
  World Frame : sm_lib/Frames and Transforms/World Frame
  B : PMIOPort  Side=Left
  Bus Element Out : Outport  VectorParamsAs1DForOutWhenUnconnected=off  PortName=Body  Element=x
  Bus Element Out1 : Outport  VectorParamsAs1DForOutWhenUnconnected=off  PortName=Body  Element=y
  Bus Element Out2 : Outport  VectorParamsAs1DForOutWhenUnconnected=off  PortName=Body  Element=z
  Bus Element Out3 : Outport  VectorParamsAs1DForOutWhenUnconnected=off  PortName=Body  Element=vx
  Bus Element Out4 : Outport  VectorParamsAs1DForOutWhenUnconnected=off  PortName=Body  Element=vy
  Bus Element Out5 : Outport  VectorParamsAs1DForOutWhenUnconnected=off  PortName=Body  Element=vz
  Bus Element Out6 : Outport  VectorParamsAs1DForOutWhenUnconnected=off  PortName=Body  Element=gx
  Bus Element Out7 : Outport  VectorParamsAs1DForOutWhenUnconnected=off  PortName=Body  Element=gy
  Bus Element Out8 : Outport  VectorParamsAs1DForOutWhenUnconnected=off  PortName=Body  Element=gz
  Bus Element Out9 : Outport  VectorParamsAs1DForOutWhenUnconnected=off  PortName=Body  Element=nRoll
  Bus Element Out10 : Outport  VectorParamsAs1DForOutWhenUnconnected=off  PortName=Body  Element=nPitch
  Bus Element Out11 : Outport  VectorParamsAs1DForOutWhenUnconnected=off  PortName=Body  Element=nYaw
  Bus Element Out12 : Outport  VectorParamsAs1DForOutWhenUnconnected=off  PortName=Body  Element=aRoll
  Bus Element Out13 : Outport  VectorParamsAs1DForOutWhenUnconnected=off  PortName=Body  Element=aPitch
  Bus Element Out14 : Outport  VectorParamsAs1DForOutWhenUnconnected=off  PortName=Body  Element=aYaw
  wires:
  PS-Simulink Converter9/1 -> Bus Element Out8/1
  PS-Simulink Converter11/1 -> Roll Pitch/1(R)
  PS-Simulink Converter6/1 -> Bus Element Out5/1
  PS-Simulink Converter7/1 -> Bus Element Out6/1
  PS-Simulink Converter2/1 -> Bus Element Out1/1
  PS-Simulink Converter8/1 -> Bus Element Out7/1
  PS-Simulink Converter5/1 -> Bus Element Out4/1
  PS-Simulink Converter3/1 -> Bus Element Out2/1
  PS-Simulink Converter1/1 -> Bus Element Out/1
  PS-Simulink Converter4/1 -> Bus Element Out3/1
  Signal Specification/1 -> Bus Element Out12/1
  Signal Specification1/1 -> Bus Element Out13/1
  Signal Specification2/1 -> Bus Element Out14/1
  Signal Specification3/1 -> Bus Element Out9/1
  Signal Specification4/1 -> Bus Element Out10/1
  Signal Specification5/1 -> Bus Element Out11/1
  Constant/1 -> Signal Specification2/1
  Constant1/1 -> Signal Specification5/1
  Roll Pitch/3(nRoll) -> Signal Specification3/1
  Roll Pitch/4(nPitch) -> Signal Specification4/1
  Roll Pitch/2(aPitch) -> Signal Specification1/1
  Roll Pitch/1(aRoll) -> Signal Specification/1
  connections:
  Transform Sensor Body/RConn5 -- PS-Simulink Converter3/LConn1
  Transform Sensor Body/RConn4 -- PS-Simulink Converter2/LConn1
  Transform Sensor Body/RConn11 -- PS-Simulink Converter9/LConn1
  Transform Sensor Body/RConn2 -- PS-Simulink Converter11/LConn1
  Transform Sensor Body/RConn7 -- PS-Simulink Converter5/LConn1
  Transform Sensor Body/RConn3 -- PS-Simulink Converter1/LConn1
  Transform Sensor Body/LConn1 -- World Frame/RConn1
  Transform Sensor Offset/LConn1 -- B/RConn1
  Transform Sensor Body/RConn10 -- PS-Simulink Converter8/LConn1
  Transform Sensor Body/RConn9 -- PS-Simulink Converter7/LConn1
  Transform Sensor Body/RConn8 -- PS-Simulink Converter6/LConn1
  Transform Sensor Body/RConn6 -- PS-Simulink Converter4/LConn1
  Transform Sensor Body/RConn1 -- Transform Sensor Offset/RConn1

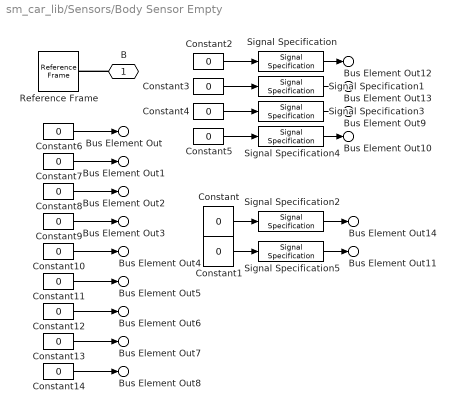
== system sm_car_lib/Sensors/Body Sensor Empty ==
  Constant{,1..14} (15 alike) : Constant  Value=0
  Reference Frame : sm_lib/Frames and Transforms/Reference Frame
  Signal Specification : SignalSpecification  Unit=rad
  Signal Specification1 : SignalSpecification  Unit=rad
  Signal Specification2 : SignalSpecification  Unit=rad
  Signal Specification3 : SignalSpecification  Unit=rad/s
  Signal Specification4 : SignalSpecification  Unit=rad/s
  Signal Specification5 : SignalSpecification  Unit=rad/s
  B : PMIOPort  Side=Left
  Bus Element Out : Outport  VectorParamsAs1DForOutWhenUnconnected=off  PortName=Body  Element=x
  Bus Element Out1 : Outport  VectorParamsAs1DForOutWhenUnconnected=off  PortName=Body  Element=y
  Bus Element Out2 : Outport  VectorParamsAs1DForOutWhenUnconnected=off  PortName=Body  Element=z
  Bus Element Out3 : Outport  VectorParamsAs1DForOutWhenUnconnected=off  PortName=Body  Element=vx
  Bus Element Out4 : Outport  VectorParamsAs1DForOutWhenUnconnected=off  PortName=Body  Element=vy
  Bus Element Out5 : Outport  VectorParamsAs1DForOutWhenUnconnected=off  PortName=Body  Element=vz
  Bus Element Out6 : Outport  VectorParamsAs1DForOutWhenUnconnected=off  PortName=Body  Element=gx
  Bus Element Out7 : Outport  VectorParamsAs1DForOutWhenUnconnected=off  PortName=Body  Element=gy
  Bus Element Out8 : Outport  VectorParamsAs1DForOutWhenUnconnected=off  PortName=Body  Element=gz
  Bus Element Out9 : Outport  VectorParamsAs1DForOutWhenUnconnected=off  PortName=Body  Element=nRoll
  Bus Element Out10 : Outport  VectorParamsAs1DForOutWhenUnconnected=off  PortName=Body  Element=nPitch
  Bus Element Out11 : Outport  VectorParamsAs1DForOutWhenUnconnected=off  PortName=Body  Element=nYaw
  Bus Element Out12 : Outport  VectorParamsAs1DForOutWhenUnconnected=off  PortName=Body  Element=aRoll
  Bus Element Out13 : Outport  VectorParamsAs1DForOutWhenUnconnected=off  PortName=Body  Element=aPitch
  Bus Element Out14 : Outport  VectorParamsAs1DForOutWhenUnconnected=off  PortName=Body  Element=aYaw
  wires:
  Constant2/1 -> Signal Specification/1
  Constant3/1 -> Signal Specification1/1
  Constant5/1 -> Signal Specification4/1
  Constant4/1 -> Signal Specification3/1
  Constant1/1 -> Signal Specification5/1
  Constant/1 -> Signal Specification2/1
  Signal Specification5/1 -> Bus Element Out11/1
  Signal Specification4/1 -> Bus Element Out10/1
  Signal Specification3/1 -> Bus Element Out9/1
  Signal Specification2/1 -> Bus Element Out14/1
  Signal Specification1/1 -> Bus Element Out13/1
  Signal Specification/1 -> Bus Element Out12/1
  Constant9/1 -> Bus Element Out3/1
  Constant6/1 -> Bus Element Out/1
  Constant8/1 -> Bus Element Out2/1
  Constant10/1 -> Bus Element Out4/1
  Constant13/1 -> Bus Element Out7/1
  Constant7/1 -> Bus Element Out1/1
  Constant12/1 -> Bus Element Out6/1
  Constant11/1 -> Bus Element Out5/1
  Constant14/1 -> Bus Element Out8/1
  connections:
  B/RConn1 -- Reference Frame/RConn1

== system sm_car_lib/Suspensions/Wheel Measurements ==
  Bus Creator : BusCreator  Inputs=2
  Calculate Camber : Subsystem
  Calculate Toe : Subsystem
  Gain2 : Gain  Gain=[1 -1 1]'
  PS-Simulink Converter1 : nesl_utility/PS-Simulink Converter  PhysicalDomain=network_engine_domain  SubClassName=ps_output  LeftPortType=input  RightPortType=output  PseudoPeriodic=off  Frequencies=[]  VectorFormat=1-D array  Unit=1  AffineConversion=off
  Reference Frame : sm_lib/Frames and Transforms/Reference Frame
  Scope : Scope
  Select z axis : Selector  NumberOfDimensions=2  InputPortWidth=2  IndexOptions=Index vector (dialog),Index vector (dialog)  Indices=[1 2 3],3  OutputSizes=1,1
  Transform Sensor1 : sm_lib/Frames and Transforms/Transform Sensor  MeasurementFrame=Base  RotationSequence=XYX  SenseAngle=off  SenseAxis=off  SenseQ=off  SenseR=on  SenseRotationSequence=off  SenseOmegaX=off  SenseOmegaY=off  SenseOmegaZ=off  SenseOmega=off  SenseQDot=off  SenseRDot=off  SenseRotationSequenceDot=off  SenseAlphaX=off  SenseAlphaY=off  SenseAlphaZ=off  SenseAlpha=off  SenseQDDot=off  SenseRDDot=off  SenseX=off  SenseY=off  SenseZ=off  SenseXYZ=off  SenseRad=off  SenseAzim=off  SenseDist=off  SenseInc=off  SenseXDot=off  SenseYDot=off  SenseZDot=off  SenseXYZDot=off  SenseRadDot=off  SenseAzimDot=off  SenseDistDot=off  SenseIncDot=off  SenseXDDot=off  SenseYDDot=off  SenseZDDot=off  SenseXYZDDot=off  SenseRadDDot=off  SenseAzimDDot=off  SenseDistDDot=off  SenseIncDDot=off
  World Frame : sm_lib/Frames and Transforms/World Frame
  Ref : PMIOPort  Side=Left
  Whl Ctr : PMIOPort  Port=2  Side=Left
  meas : Outport  VectorParamsAs1DForOutWhenUnconnected=off
  wires:
  Calculate Toe/1(Toe) -> Bus Creator/1  "aToe"
  Calculate Camber/1(Camber) -> Bus Creator/2  "aCamber"
  Gain2/1 -> Calculate Camber/1(uvec spin axis), Calculate Toe/1(uvec spin axis)
  PS-Simulink Converter1/1 -> Select z axis/1
  Select z axis/1 -> Gain2/1, Scope/1  "uvec spin axis"
  Bus Creator/1 -> meas/1  "Whl"
  connections:
  Transform Sensor1/LConn1 -- World Frame/RConn1
  PS-Simulink Converter1/LConn1 -- Transform Sensor1/RConn2
  Transform Sensor1/RConn1 -- Whl Ctr/RConn1
  Ref/RConn1 -- Reference Frame/RConn1

== system sm_car_lib/Tires/Ground ==
  gz : Inport
  uvec : Inport  Port=2
  TyreScaling FL : Inport  Port=3
  TyreScaling FR : Inport  Port=4
  TyreScaling RL : Inport  Port=5
  TyreScaling RR : Inport  Port=6
  Bus Creator{,1..3} (4 alike) : BusCreator  Inputs=3
  Bus Selector : BusSelector  OutputSignals=L1,R1,L2,R2
  Bus Selector1 : BusSelector  OutputSignals=L1,R1,L2,R2
  Gain{,1..7} (8 alike) : Gain
  Signal Specification1 : SignalSpecification  Unit=m
  L1 : Outport  VectorParamsAs1DForOutWhenUnconnected=off
  R1 : Outport  Port=2  VectorParamsAs1DForOutWhenUnconnected=off
  L2 : Outport  Port=3  VectorParamsAs1DForOutWhenUnconnected=off
  R2 : Outport  Port=4  VectorParamsAs1DForOutWhenUnconnected=off
  wires:
  Bus Creator/1 -> L1/1  "L1"
  Bus Creator1/1 -> R1/1  "R1"
  Gain1/1 -> Bus Creator1/1  "gz"
  TyreScaling FL/1 -> Bus Creator/3  "TyreScaling"
  Bus Creator3/1 -> R2/1  "R2"
  gz/1 -> Signal Specification1/1
  Gain3/1 -> Bus Creator3/1  "gz"
  Bus Creator2/1 -> L2/1  "L2"
  Signal Specification1/1 -> Bus Selector/1
  Gain2/1 -> Bus Creator2/1  "gz"
  TyreScaling FR/1 -> Bus Creator1/3  "TyreScaling"
  TyreScaling RL/1 -> Bus Creator2/3  "TyreScaling"
  TyreScaling RR/1 -> Bus Creator3/3  "TyreScaling"
  Bus Selector/1 -> Gain/1  "<L1>"
  Gain/1 -> Bus Creator/1  "gz"
  Bus Selector/2 -> Gain1/1  "<R1>"
  Bus Selector/3 -> Gain2/1  "<L2>"
  Bus Selector/4 -> Gain3/1  "<R2>"
  uvec/1 -> Bus Selector1/1
  Bus Selector1/1 -> Gain4/1  "<L1>"
  Bus Selector1/2 -> Gain5/1  "<R1>"
  Bus Selector1/3 -> Gain6/1  "<L2>"
  Bus Selector1/4 -> Gain7/1  "<R2>"
  Gain4/1 -> Bus Creator/2  "uvec"
  Gain5/1 -> Bus Creator1/2  "uvec"
  Gain6/1 -> Bus Creator2/2  "uvec"
  Gain7/1 -> Bus Creator3/2  "uvec"

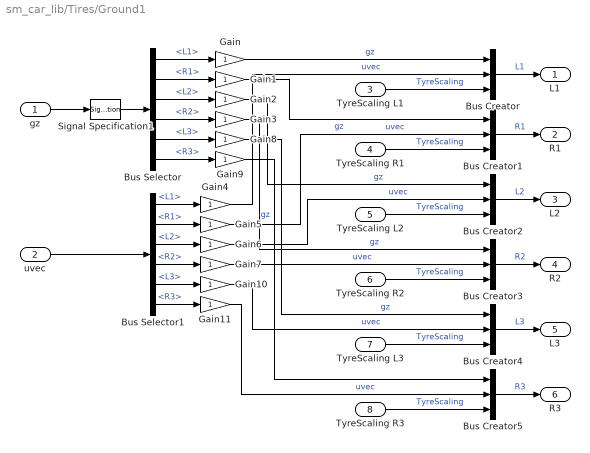
== system sm_car_lib/Tires/Ground1 ==
  gz : Inport
  uvec : Inport  Port=2
  TyreScaling L1 : Inport  Port=3
  TyreScaling R1 : Inport  Port=4
  TyreScaling L2 : Inport  Port=5
  TyreScaling R2 : Inport  Port=6
  TyreScaling L3 : Inport  Port=7
  TyreScaling R3 : Inport  Port=8
  Bus Creator{,1..5} (6 alike) : BusCreator  Inputs=3
  Bus Selector : BusSelector  OutputSignals=L1,R1,L2,R2,L3,R3
  Bus Selector1 : BusSelector  OutputSignals=L1,R1,L2,R2,L3,R3
  Gain{,1..11} (12 alike) : Gain
  Signal Specification1 : SignalSpecification  Unit=m
  L1 : Outport  VectorParamsAs1DForOutWhenUnconnected=off
  R1 : Outport  Port=2  VectorParamsAs1DForOutWhenUnconnected=off
  L2 : Outport  Port=3  VectorParamsAs1DForOutWhenUnconnected=off
  R2 : Outport  Port=4  VectorParamsAs1DForOutWhenUnconnected=off
  L3 : Outport  Port=5  VectorParamsAs1DForOutWhenUnconnected=off
  R3 : Outport  Port=6  VectorParamsAs1DForOutWhenUnconnected=off
  wires:
  Gain7/1 -> Bus Creator3/2  "uvec"
  Gain6/1 -> Bus Creator2/2  "uvec"
  Gain5/1 -> Bus Creator1/2  "uvec"
  Gain4/1 -> Bus Creator/2  "uvec"
  Bus Selector1/4 -> Gain7/1  "<R2>"
  Bus Selector1/3 -> Gain6/1  "<L2>"
  Bus Selector1/2 -> Gain5/1  "<R1>"
  Bus Selector1/1 -> Gain4/1  "<L1>"
  uvec/1 -> Bus Selector1/1
  Bus Selector/4 -> Gain3/1  "<R2>"
  Bus Selector/3 -> Gain2/1  "<L2>"
  Bus Selector/2 -> Gain1/1  "<R1>"
  Gain/1 -> Bus Creator/1  "gz"
  Bus Selector/1 -> Gain/1  "<L1>"
  TyreScaling R2/1 -> Bus Creator3/3  "TyreScaling"
  TyreScaling L2/1 -> Bus Creator2/3  "TyreScaling"
  TyreScaling R1/1 -> Bus Creator1/3  "TyreScaling"
  Gain2/1 -> Bus Creator2/1  "gz"
  Signal Specification1/1 -> Bus Selector/1
  Bus Creator2/1 -> L2/1  "L2"
  Gain3/1 -> Bus Creator3/1  "gz"
  gz/1 -> Signal Specification1/1
  Bus Creator3/1 -> R2/1  "R2"
  TyreScaling L1/1 -> Bus Creator/3  "TyreScaling"
  Gain1/1 -> Bus Creator1/1  "gz"
  Bus Creator1/1 -> R1/1  "R1"
  Bus Creator/1 -> L1/1  "L1"
  Bus Creator5/1 -> R3/1  "R3"
  Gain9/1 -> Bus Creator5/1  "gz"
  Bus Creator4/1 -> L3/1  "L3"
  Gain8/1 -> Bus Creator4/1  "gz"
  TyreScaling L3/1 -> Bus Creator4/3  "TyreScaling"
  TyreScaling R3/1 -> Bus Creator5/3  "TyreScaling"
  Gain10/1 -> Bus Creator4/2  "uvec"
  Gain11/1 -> Bus Creator5/2  "uvec"
  Bus Selector1/5 -> Gain10/1  "<L3>"
  Bus Selector1/6 -> Gain11/1  "<R3>"
  Bus Selector/5 -> Gain8/1  "<L3>"
  Bus Selector/6 -> Gain9/1  "<R3>"
